simulink model "model1"  (R2020b)
settings: Solver=VariableStepAuto  StartTime=0.0  StopTime=10.0  MaxStep=0.001  RelTol=1e-3
values from neighbouring files (symbols this model uses):
  b = 50    [values.m]
  k1 = 50    [values.m]
  k12 = 9500    [values.m]
  m1 = 100    [values.m]
  m2 = 95    [values.m]
settings Model: Creator=Abhinav dixit  LastModifiedBy=Abhinav dixit

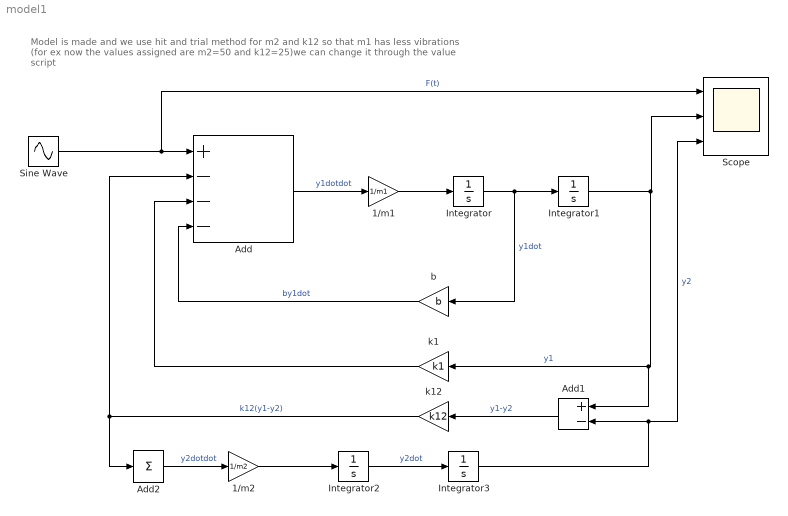
== system model1 ==
  note: Model is made and we use hit and trial method for m2 and k12 so that m1 has less vibrations (for ex now the values assigned are m2=50 and k12=25)we can change it through the value script
  1/m1 : Gain  Gain=1/m1
  1/m2 : Gain  Gain=1/m2
  Add : Sum  Inputs=+---
  Add1 : Sum  Inputs=+-
  Add2 : Sum  Inputs=+
  Integrator{,1..3} (4 alike) : Integrator
  Scope : Scope  NumInputPorts=3
  Sine Wave : Sin  Amplitude=2  Frequency=10  SampleTime=0
  b : Gain  Gain=b
  k1 : Gain  Gain=k1
  k12 : Gain  Gain=k12
  wires:
  Sine Wave/1 -> Scope/1, Add/1  "F(t)"
  Add/1 -> 1/m1/1  "y1dotdot"
  Integrator/1 -> b/1, Integrator1/1  "y1dot"
  1/m1/1 -> Integrator/1
  Integrator1/1 -> Add1/1, k1/1, Scope/2  "y1"
  b/1 -> Add/4  "by1dot"
  k1/1 -> Add/3
  Add1/1 -> k12/1  "y1-y2"
  k12/1 -> Add2/1, Add/2  "k12(y1-y2)"
  1/m2/1 -> Integrator2/1
  Integrator2/1 -> Integrator3/1  "y2dot"
  Integrator3/1 -> Scope/3, Add1/2  "y2"
  Add2/1 -> 1/m2/1  "y2dotdot"
